simulink model "Lab3_Q2"  (R2020b)
settings: Solver=VariableStepAuto  StartTime=0.0  StopTime=10.0  RelTol=1e-3
settings Model: Creator=kushagrakhatwani  LastModifiedBy=kushagrakhatwani

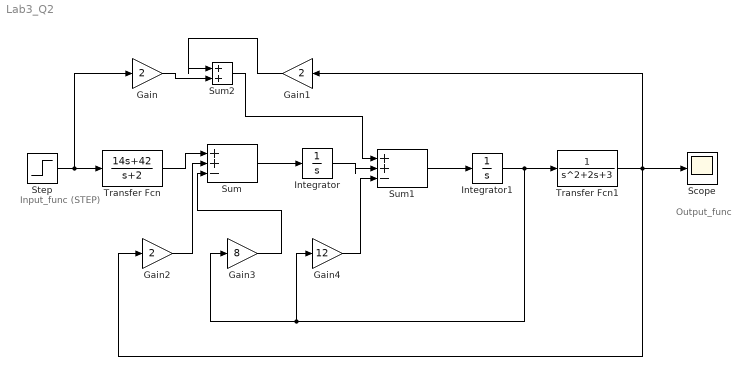
== system Lab3_Q2 ==
  note: Output_func
  note: Input_func
      | (STEP)
  Gain : Gain  Gain=2
  Gain1 : Gain  Gain=2
  Gain2 : Gain  Gain=2
  Gain3 : Gain  Gain=8
  Gain4 : Gain  Gain=12
  Integrator : Integrator
  Integrator1 : Integrator
  Scope : Scope
  Step : Step  Time=0  SampleTime=0
  Sum : Sum  Inputs=|++-
  Sum1 : Sum  Inputs=|++-
  Sum2 : Sum  Inputs=|++
  Transfer Fcn : TransferFcn  Numerator=[14 42]  Denominator=[1 2]
  Transfer Fcn1 : TransferFcn  Denominator=[1 2 3]
  wires:
  Step/1 -> Gain/1, Transfer Fcn/1
  Sum/1 -> Integrator/1
  Integrator/1 -> Sum1/2
  Sum1/1 -> Integrator1/1
  Integrator1/1 -> Gain4/1, Gain3/1, Transfer Fcn1/1
  Gain1/1 -> Sum2/1
  Transfer Fcn1/1 -> Scope/1, Gain2/1, Gain1/1
  Sum2/1 -> Sum1/1
  Gain2/1 -> Sum/2
  Transfer Fcn/1 -> Sum/1
  Gain3/1 -> Sum/3
  Gain4/1 -> Sum1/3
  Gain/1 -> Sum2/2
